simulink model "Ejer14_RolloPapel"  (R2023b)
settings: Solver=FixedStepAuto  StartTime=0.0  StopTime=1000  FixedStep=1  RelTol=1e-3
settings Model: Creator=alfre  LastModifiedBy=alfre

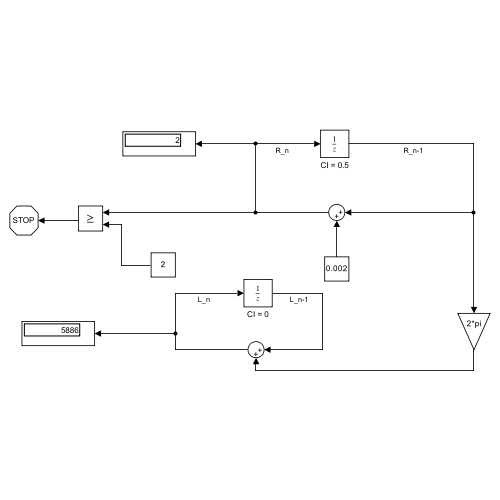
[thumbnail: Simulink's stored preview of the top-level diagram]
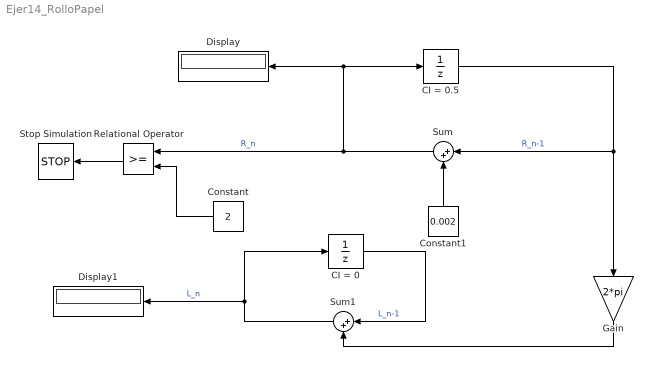
== system Ejer14_RolloPapel ==
  CI = 0 : UnitDelay  SampleTime=-1  HasFrameUpgradeWarning=on
  CI = 0.5 : UnitDelay  InitialCondition=0.5  SampleTime=-1  HasFrameUpgradeWarning=on
  Constant : Constant  Value=2
  Constant1 : Constant  Value=0.002
  Display : Display
  Display1 : Display
  Gain : Gain  Gain=2*pi
  Relational Operator : RelationalOperator  OutDataTypeStr=boolean  RndMeth=Simplest  InputSameDT=off
  Stop Simulation : Stop
  Sum : Sum  Inputs=|++
  Sum1 : Sum  Inputs=|++
  wires:
  Relational Operator/1 -> Stop Simulation/1
  CI = 0.5/1 -> Gain/1, Sum/1  "R_n-1"
  Sum/1 -> Relational Operator/1, CI = 0.5/1, Display/1  "R_n"
  Constant/1 -> Relational Operator/2
  Constant1/1 -> Sum/2
  Gain/1 -> Sum1/2
  CI = 0/1 -> Sum1/1  "L_n-1"
  Sum1/1 -> CI = 0/1, Display1/1  "L_n"
